simulink model "sixDOF6"  (R2024a)
settings: Solver=VariableStepAuto  StartTime=0.0  StopTime=30  MinStep=0.001  RelTol=1e-3
PreLoadFcn:
  | load("C:\Users\craig\OneDrive\Desktop\Matlab\TVC\Workspaces\rocketProps.mat");
undefined symbols (not defined in the file): magnitude, thrust, time
libraries: simulink x2, sharedtransform x2, aerolibanim x1, vrlib x1
settings Model: NumberOfSteps=100  Creator=craig  LastModifiedBy=craig
settings SolverCC: MaxConsecutiveMinStep=2
settings DebuggingCC: UnderSpecifiedDataTypeMsg=warning  UnderSpecifiedDimensionMsg=warning

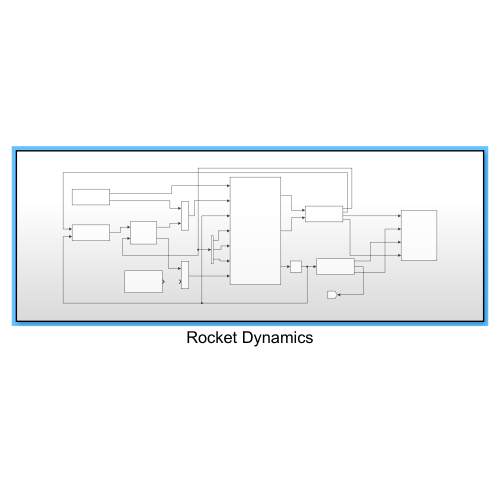
[thumbnail: Simulink's stored preview of the top-level diagram]
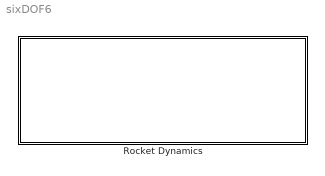
== system sixDOF6 ==
  Rocket Dynamics : Subsystem

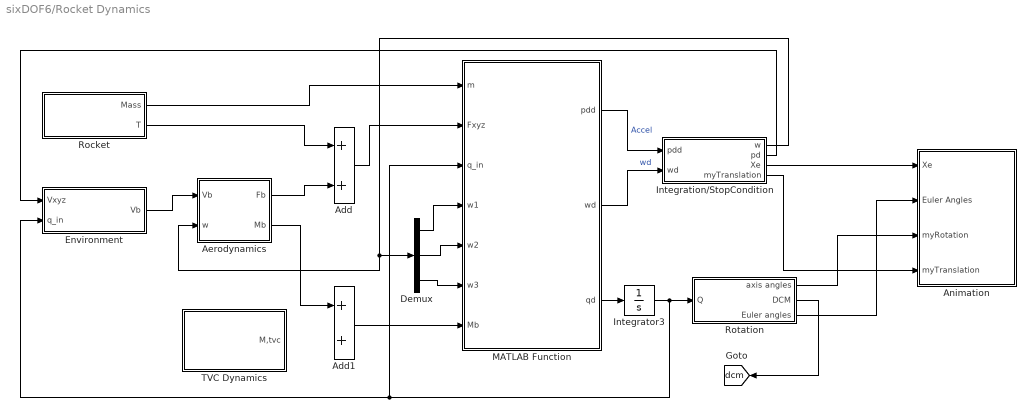
== system sixDOF6/Rocket Dynamics ==
  Add : Sum
  Add1 : Sum
  Aerodynamics : Subsystem
  Animation : Subsystem
  Demux : Demux  Outputs=3
  Environment : Subsystem
  Integration/StopCondition : Subsystem
  Integrator3 : Integrator  InitialCondition=[1; 0; 0; 0]
  MATLAB Function : MATLAB Function  TreatAsAtomicUnit=on
  Rocket : Subsystem
  Rotation : Subsystem
  TVC Dynamics : Subsystem
  tag scope: dcm=global
  wires:
  Integrator3/1 -> MATLAB Function/3(q_in), Environment/2(q_in), Rotation/1(Q)
  Add/1 -> MATLAB Function/2(Fxyz)
  Demux/1 -> MATLAB Function/4(w1)
  Environment/1("Vb ") -> Aerodynamics/1(Vb)
  Demux/3 -> MATLAB Function/6(w3)
  Aerodynamics/2(Mb) -> Add1/1
  Demux/2 -> MATLAB Function/5(w2)
  MATLAB Function/3(qd) -> Integrator3/1
  Rocket/2(T) -> Add/1
  Rocket/1(Mass) -> MATLAB Function/1(m)
  Aerodynamics/1(Fb) -> Add/2
  Rotation/2(DCM) -> [dcm]
  Add1/1 -> MATLAB Function/7(Mb)
  MATLAB Function/2(wd) -> Integration/StopCondition/2(wd)  "wd"
  Integration/StopCondition/1(w) -> Aerodynamics/2(w), Demux/1
  MATLAB Function/1(pdd) -> Integration/StopCondition/1(pdd)  "Accel"
  Integration/StopCondition/2(pd) -> Environment/1(Vxyz)
  Integration/StopCondition/3(Xe) -> Animation/1(Xe)
  Rotation/3(Euler angles) -> Animation/2(Euler Angles)
  Rotation/1(axis angles) -> Animation/3(myRotation)
  Integration/StopCondition/4(myTranslation) -> Animation/4(myTranslation)

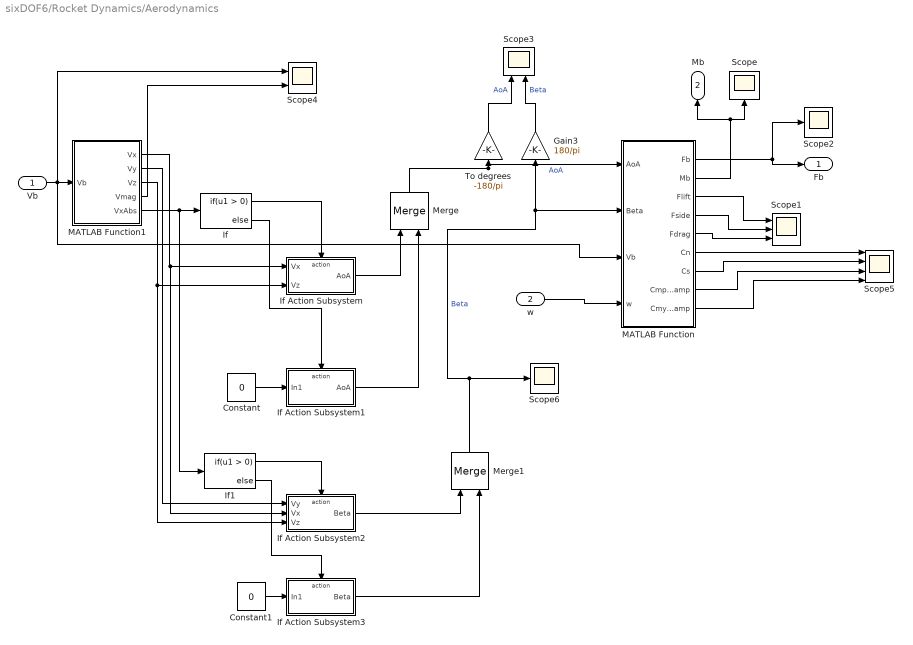
== system sixDOF6/Rocket Dynamics/Aerodynamics ==
  Vb : Inport
  w : Inport  Port=2
  Constant : Constant  Value=0
  Constant1 : Constant  Value=0
  Gain3 : Gain  Gain=180/pi
  If : If
  If Action Subsystem : Subsystem  TreatAsAtomicUnit=on
  If Action Subsystem1 : Subsystem  TreatAsAtomicUnit=on
  If Action Subsystem2 : Subsystem  TreatAsAtomicUnit=on
  If Action Subsystem3 : Subsystem  TreatAsAtomicUnit=on
  If1 : If
  MATLAB Function : MATLAB Function  TreatAsAtomicUnit=on
  MATLAB Function1 : MATLAB Function  TreatAsAtomicUnit=on
  Merge : Merge
  Merge1 : Merge
  Scope : Scope
  Scope1 : Scope  NumInputPorts=3
  Scope2 : Scope
  Scope3 : Scope  NumInputPorts=2
  Scope4 : Scope  NumInputPorts=2
  Scope5 : Scope  NumInputPorts=4
  Scope6 : Scope
  To degrees : Gain  Gain=-180/pi
  Fb : Outport
  Mb : Outport  Port=2
  wires:
  MATLAB Function/3(Flift) -> Scope1/1
  MATLAB Function/2(Mb) -> Scope/1, Mb/1
  MATLAB Function/1(Fb) -> Scope2/1, Fb/1
  MATLAB Function/5(Fdrag) -> Scope1/3
  Vb/1 -> Scope4/1, MATLAB Function/3(Vb), MATLAB Function1/1(Vb)
  If/2 -> If Action Subsystem1/Action
  Constant/1 -> If Action Subsystem1/1(In1)
  MATLAB Function1/1(Vx) -> If Action Subsystem2/2(Vx), If Action Subsystem/1(Vx)
  MATLAB Function1/3(Vz) -> If Action Subsystem2/3(Vz), If Action Subsystem/2(Vz)
  If/1 -> If Action Subsystem/Action
  If Action Subsystem/1(AoA) -> Merge/1
  If Action Subsystem1/1(AoA) -> Merge/2
  MATLAB Function1/2(Vy) -> If Action Subsystem2/1(Vy)
  Constant1/1 -> If Action Subsystem3/1(In1)
  If Action Subsystem2/1(Beta) -> Merge1/1
  If Action Subsystem3/1(Beta) -> Merge1/2
  If1/2 -> If Action Subsystem3/Action
  If1/1 -> If Action Subsystem2/Action
  MATLAB Function/4(Fside) -> Scope1/2
  Merge1/1 -> Scope6/1, Gain3/1, MATLAB Function/2(Beta)  "Beta"
  Merge/1 -> To degrees/1, MATLAB Function/1(AoA)  "AoA"
  MATLAB Function/6(Cn) -> Scope5/1
  MATLAB Function/7(Cs) -> Scope5/2
  Gain3/1 -> Scope3/2  "Beta"
  To degrees/1 -> Scope3/1  "AoA"
  MATLAB Function1/4(Vmag) -> Scope4/2
  MATLAB Function1/5(VxAbs) -> If1/1, If/1
  w/1 -> MATLAB Function/4(w)
  MATLAB Function/8(CmpDamp) -> Scope5/3
  MATLAB Function/9(CmyDamp) -> Scope5/4

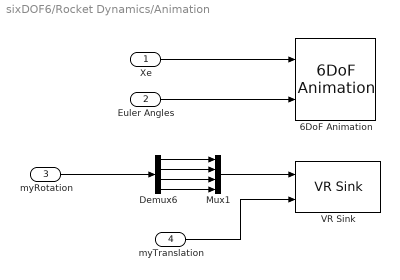
== system sixDOF6/Rocket Dynamics/Animation ==
  Xe : Inport
  Euler Angles : Inport  Port=2
  myRotation : Inport  Port=3
  myTranslation : Inport  Port=4
  6DoF Animation : aerolibanim/6DoF Animation  u1=[0 4000 -2000 2000 -5000 -3000]  u2=0.1  u3=100  u4=[4000 0 -5000]  u5=Fixed position  u6=[2000 500 -3150]  u7=10  u8=on
  Demux6 : Demux
  Mux1 : Mux
  VR Sink : vrlib/VR Sink  InstantiateOnLoad=on  SampleTime=0.1  ViewEnable=on  RemoteChange=off  RemoteView=off  FieldsWritten=MyTransform.rotation.4.1.1.double#MyTransform.translation.3.1.1.double  WorldFileName=C:\Users\craig\OneDrive\Desktop\Matlab\TVC\Animations\BestViewpoint.wrl  AutoView=off  VideoDimensions=[]  AllowVariableSize=off
  wires:
  Xe/1 -> 6DoF Animation/1
  Demux6/1 -> Mux1/1
  Demux6/3 -> Mux1/3
  myTranslation/1 -> VR Sink/2
  Demux6/2 -> Mux1/2
  Mux1/1 -> VR Sink/1
  myRotation/1 -> Demux6/1
  Demux6/4 -> Mux1/4
  Euler Angles/1 -> 6DoF Animation/2

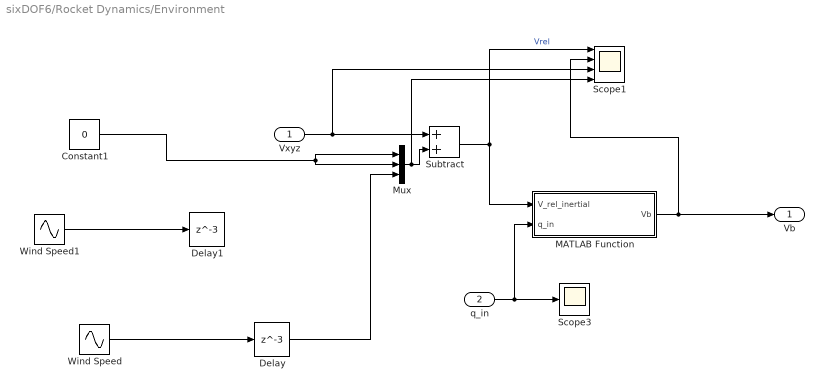
== system sixDOF6/Rocket Dynamics/Environment ==
  Vxyz : Inport
  q_in : Inport  Port=2
  Constant1 : Constant  Value=0
  Delay : Delay  DelayLength=3
  Delay1 : Delay  DelayLength=3
  MATLAB Function : MATLAB Function  TreatAsAtomicUnit=on
  Mux : Mux  Inputs=3
  Scope1 : Scope  NumInputPorts=4
  Scope3 : Scope
  Subtract : Sum
  Wind Speed : Sin  Amplitude=0.5  Bias=5  Frequency=2*pi*0.25  SampleTime=0
  Wind Speed1 : Sin  Amplitude=0.5  Bias=5  Frequency=2*pi*0.25  SampleTime=0
  "Vb " : Outport
  wires:
  Subtract/1 -> Scope1/1, MATLAB Function/1(V_rel_inertial)  "Vrel"
  Vxyz/1 -> Subtract/1, Scope1/3
  MATLAB Function/1(Vb) -> "Vb "/1, Scope1/2
  Constant1/1 -> Mux/1, Mux/2
  q_in/1 -> MATLAB Function/2(q_in), Scope3/1
  Mux/1 -> Scope1/4, Subtract/2
  Wind Speed1/1 -> Delay1/1
  Wind Speed/1 -> Delay/1
  Delay/1 -> Mux/3

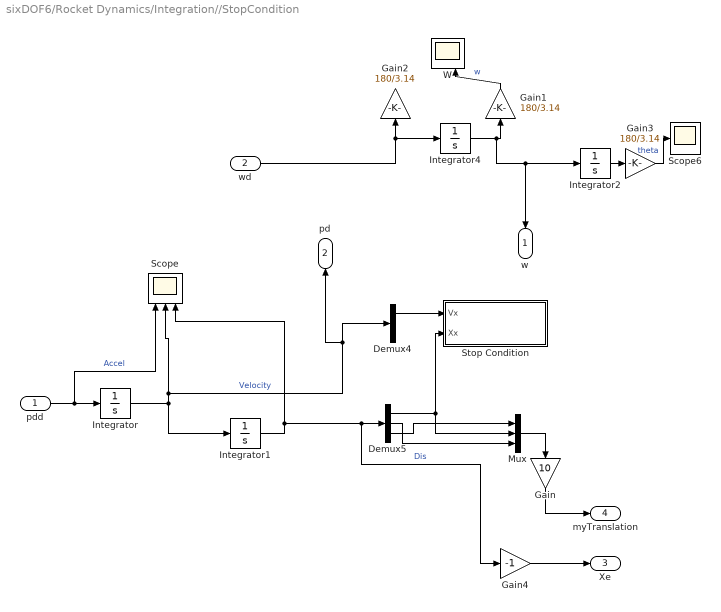
== system sixDOF6/Rocket Dynamics/Integration//StopCondition ==
  pdd : Inport
  wd : Inport  Port=2
  Demux4 : Demux  Outputs=3
  Demux5 : Demux  Outputs=3
  Gain : Gain  Gain=10
  Gain1 : Gain  Gain=180/3.14
  Gain2 : Gain  Gain=180/3.14
  Gain3 : Gain  Gain=180/3.14
  Gain4 : Gain  Gain=-1
  Integrator{,1..2,4} (4 alike) : Integrator  InitialCondition=[0; 0; 0]
  Mux : Mux  Inputs=3
  Scope : Scope  NumInputPorts=3
  Scope6 : Scope
  Stop Condition : Subsystem
  W : Scope  NumInputPorts=2
  w : Outport
  pd : Outport  Port=2
  Xe : Outport  Port=3
  myTranslation : Outport  Port=4
  wires:
  wd/1 -> Integrator4/1, Gain2/1
  Integrator2/1 -> Gain3/1
  Integrator4/1 -> w/1, Integrator2/1, Gain1/1
  Gain1/1 -> W/2  "w"
  Gain3/1 -> Scope6/1  "theta"
  Integrator/1 -> Integrator1/1, Demux4/1, pd/1, Scope/2  "Velocity"
  Demux5/3 -> Mux/1
  Demux5/2 -> Mux/3
  Demux4/1 -> Stop Condition/1(Vx)
  pdd/1 -> Scope/1, Integrator/1  "Accel"
  Gain4/1 -> Xe/1
  Integrator1/1 -> Scope/3, Gain4/1, Demux5/1  "Dis"
  Gain/1 -> myTranslation/1
  Mux/1 -> Gain/1
  Demux5/1 -> Stop Condition/2(Xx), Mux/2

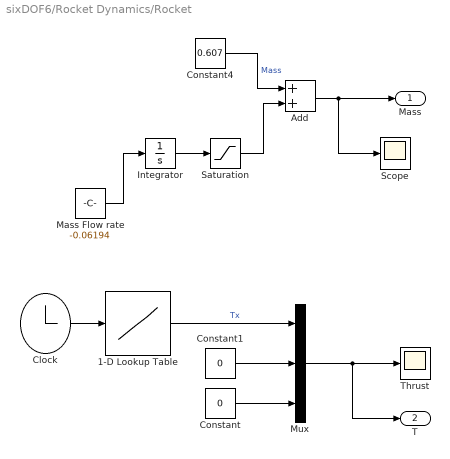
== system sixDOF6/Rocket Dynamics/Rocket ==
  1-D Lookup Table : Lookup_n-D  NumberOfTableDimensions=1  BreakpointsForDimension1=time  Table=thrust  TableMin=[0]  TableDataTypeStr=Inherit: Inherit from 'Table data'  ExtrapMethod=Clip  UseLastTableValue=on  InternalRulePriority=Speed  RndMeth=Simplest
  Add : Sum
  Clock : Clock
      settings: Decimation=100
  Constant : Constant  Value=0
  Constant1 : Constant  Value=0
  Constant4 : Constant  Value=0.607
  Integrator : Integrator  InitialCondition=0.188
  Mass Flow rate : Constant  Value=-0.06194
  Mux : Mux  Inputs=3
  Saturation : Saturate  LowerLimit=0.105
  Scope : Scope
  Thrust : Scope
  Mass : Outport
  T : Outport  Port=2
  wires:
  Clock/1 -> 1-D Lookup Table/1
  Constant1/1 -> Mux/2
  Mux/1 -> T/1, Thrust/1
  Constant4/1 -> Add/1  "Mass"
  Add/1 -> Scope/1, Mass/1
  1-D Lookup Table/1 -> Mux/1  "Tx"
  Constant/1 -> Mux/3
  Mass Flow rate/1 -> Integrator/1
  Integrator/1 -> Saturation/1
  Saturation/1 -> Add/2

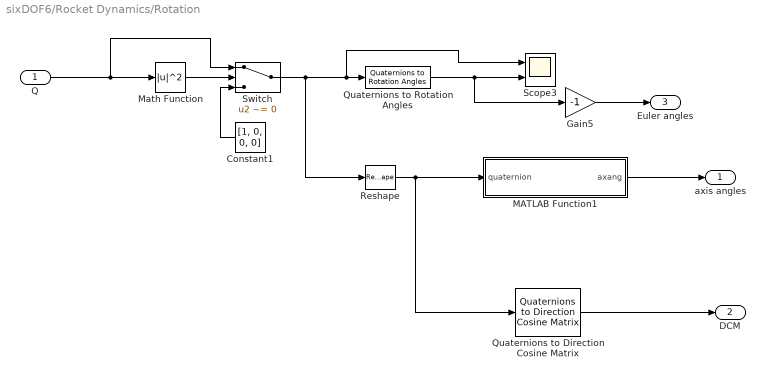
== system sixDOF6/Rocket Dynamics/Rotation ==
  Q : Inport
  Constant1 : Constant  Value=[1, 0, 0, 0]
  Gain5 : Gain  Gain=-1
  MATLAB Function1 : MATLAB Function  TreatAsAtomicUnit=on
  Math Function : Math  Operator=magnitude^2
  Quaternions to Direction Cosine Matrix : sharedtransform/Quaternions to  Direction Cosine Matrix  aMode=aMode
      settings: LibrarySourceBlock=|
      | aerolibtransform2/Quaternions to
      | Direction Cosine Matrix
  Quaternions to Rotation Angles : sharedtransform/Quaternions to Rotation Angles  rotationOrder=XYZ  aMode=aMode
  Reshape : Reshape  OutputDimensionality=Customize  OutputDimensions=[1,4]
  Scope3 : Scope  NumInputPorts=2
  Switch : Switch  Criteria=u2 ~= 0  SaturateOnIntegerOverflow=off  InputSameDT=off
  axis angles : Outport
  DCM : Outport  Port=2
  Euler angles : Outport  Port=3
  wires:
  Constant1/1 -> Switch/3
  Quaternions to Rotation Angles/1 -> Gain5/1, Scope3/2
  Switch/1 -> Reshape/1, Scope3/1, Quaternions to Rotation Angles/1
  Math Function/1 -> Switch/2
  Q/1 -> Switch/1, Math Function/1
  MATLAB Function1/1(axang) -> axis angles/1
  Reshape/1 -> Quaternions to Direction Cosine Matrix/1, MATLAB Function1/1(quaternion)
  Quaternions to Direction Cosine Matrix/1 -> DCM/1
  Gain5/1 -> Euler angles/1

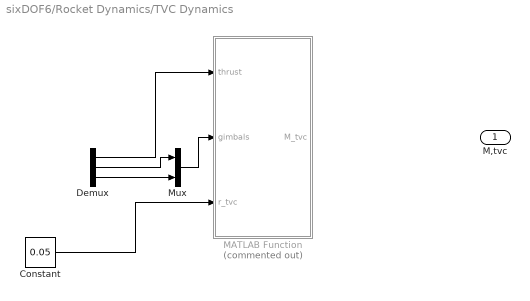
== system sixDOF6/Rocket Dynamics/TVC Dynamics ==
  Constant : Constant  Value=0.05
  Demux : Demux  Outputs=3
  MATLAB Function : MATLAB Function  Commented=on  TreatAsAtomicUnit=on
  Mux : Mux  Inputs=2
  M,tvc : Outport
  wires:
  Demux/1 -> MATLAB Function/1(thrust)
  Demux/2 -> Mux/1
  Demux/3 -> Mux/2
  Mux/1 -> MATLAB Function/2(gimbals)
  Constant/1 -> MATLAB Function/3(r_tvc)

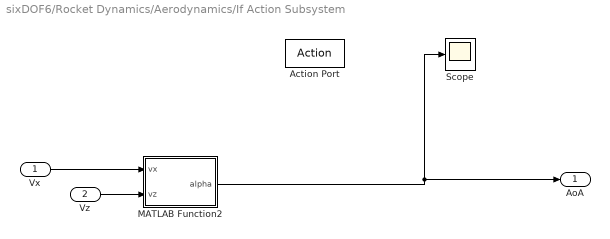
== system sixDOF6/Rocket Dynamics/Aerodynamics/If Action Subsystem ==
  Vx : Inport
  Vz : Inport  Port=2
  Action Port : ActionPort  ActionPortLabel=if(u1 > 0)
  MATLAB Function2 : MATLAB Function  TreatAsAtomicUnit=on
  Scope : Scope
  AoA : Outport
  wires:
  MATLAB Function2/1(alpha) -> Scope/1, AoA/1
  Vx/1 -> MATLAB Function2/1(vx)
  Vz/1 -> MATLAB Function2/2(vz)

== system sixDOF6/Rocket Dynamics/Aerodynamics/If Action Subsystem1 ==
  In1 : Inport
  Action Port : ActionPort  ActionPortLabel=else
  AoA : Outport
  wires:
  In1/1 -> AoA/1

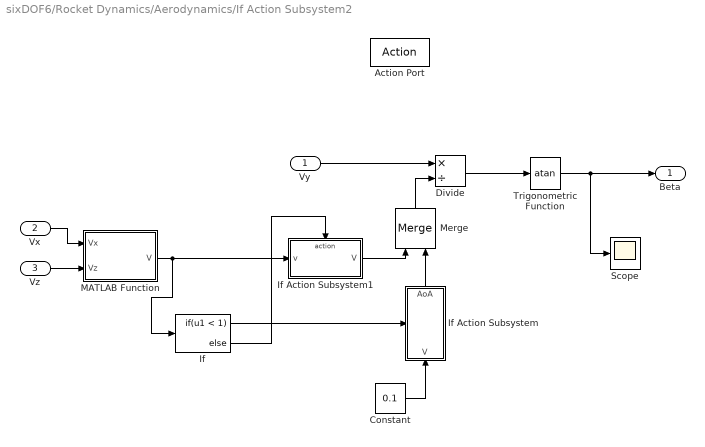
== system sixDOF6/Rocket Dynamics/Aerodynamics/If Action Subsystem2 ==
  Vy : Inport
  Vx : Inport  Port=2
  Vz : Inport  Port=3
  Action Port : ActionPort  ActionPortLabel=if(u1 > 0)
  Constant : Constant  Value=0.1
  Divide : Product  Inputs=*/
  If : If  IfExpression=u1 < 1
  If Action Subsystem : Subsystem  TreatAsAtomicUnit=on
  If Action Subsystem1 : Subsystem  TreatAsAtomicUnit=on
  MATLAB Function : MATLAB Function  TreatAsAtomicUnit=on
  Merge : Merge
  Scope : Scope
  Trigonometric Function : Trigonometry  Operator=atan
  Beta : Outport
  wires:
  Vx/1 -> MATLAB Function/1(Vx)
  Vz/1 -> MATLAB Function/2(Vz)
  Divide/1 -> Trigonometric Function/1
  Vy/1 -> Divide/1
  Constant/1 -> If Action Subsystem/1(V)
  Trigonometric Function/1 -> Scope/1, Beta/1
  If/1 -> If Action Subsystem/Action
  If Action Subsystem/1(AoA) -> Merge/2
  If/2 -> If Action Subsystem1/Action
  If Action Subsystem1/1(V) -> Merge/1
  Merge/1 -> Divide/2
  MATLAB Function/1(V) -> If/1, If Action Subsystem1/1(v)

== system sixDOF6/Rocket Dynamics/Aerodynamics/If Action Subsystem3 ==
  In1 : Inport
  Action Port : ActionPort  ActionPortLabel=else
  Beta : Outport
  wires:
  In1/1 -> Beta/1

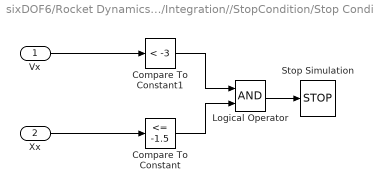
== system sixDOF6/Rocket Dynamics/Integration//StopCondition/Stop Condition ==
  Vx : Inport
  Xx : Inport  Port=2
  Compare To Constant : simulink/Logic and Bit Operations/Compare To Constant  relop=<=  const=-1.5  OutDataTypeStr=boolean
  Compare To Constant1 : simulink/Logic and Bit Operations/Compare To Constant  relop=<  const=-3  OutDataTypeStr=boolean
  Logical Operator : Logic  AllPortsSameDT=off  OutDataTypeStr=boolean
  Stop Simulation : Stop
  wires:
  Compare To Constant/1 -> Logical Operator/2
  Vx/1 -> Compare To Constant1/1
  Xx/1 -> Compare To Constant/1
  Compare To Constant1/1 -> Logical Operator/1
  Logical Operator/1 -> Stop Simulation/1

== system sixDOF6/Rocket Dynamics/Aerodynamics/If Action Subsystem2/If Action Subsystem ==
  V : Inport
  Action Port : ActionPort  ActionPortLabel=if(u1 < 1)
  AoA : Outport
  wires:
  V/1 -> AoA/1

== system sixDOF6/Rocket Dynamics/Aerodynamics/If Action Subsystem2/If Action Subsystem1 ==
  v : Inport
  Action Port : ActionPort  ActionPortLabel=else
  V : Outport
  wires:
  v/1 -> V/1

== matlab function sixDOF6/Rocket Dynamics/Aerodynamics/If Action Subsystem2/MATLAB Function ==
  data: Vx input; V output; Vz input
function V = fcn(Vx, Vz)

Vyz = [Vx; Vz];
V = norm(Vyz);

== matlab function sixDOF6/Rocket Dynamics/TVC Dynamics/MATLAB Function ==
  data: thrust input; M_tvc output; gimbals input; r_tvc input
function M_tvc = TVC_Controller(thrust, gimbals, r_tvc)


%TVC_Controller: Computes the thrust vector and the resulting moment

theta = gimbals(1);
psi = gimbals(2);

    % Define the thrust vector in the body frame
    TVC_body = thrust * [cos(theta) * cos(psi);  sin(psi); sin(theta)];
    
    % Calculate the moment arm (r_tvc cross T_body)
    M_tvc = cross(r_tvc, TVC_body);
    

end

== matlab function sixDOF6/Rocket Dynamics/Aerodynamics/If Action Subsystem/MATLAB Function2 ==
  data: vx input; alpha output; vz input
function alpha = fcn(vx, vz)

%if abs(vx) < 5
 %   alpha = 0;
%else
    alpha = atan2(vz, vx);
end

== matlab function sixDOF6/Rocket Dynamics/MATLAB Function ==
  data: m input; Fxyz input; q_in input size=4; w1 input; w2 input; w3 input; Mb input; pdd output size=[3,1]; wd output size=[3,1]; qd output
function [pdd, wd, qd] = EOM(m, Fxyz, q_in, w1, w2, w3, Mb)

q_in = q_in / norm(q_in); %normalise quaternion
Ix=0.00083;
Iy=0.00073;
Iz=0.00073;
g=9.81;
wx=w1;
wy=w2;
wz=w3;
w=[w1;w2;w3];

%Angular accelerations using newtons 2nd law for rotations in body frame
wxd = (1/Ix) * (Mb(1) + (Iy - Iz) * wy * wz);
wyd = (1/Iy) * (Mb(2) + (Iz - Ix) * wx * wz);
wzd = (1/Iz) * (Mb(3) + (Ix - Iy) * wx * wy);
wd =[wxd;wyd;wzd];


%update quaternion to reflect attitude change using formula for RoC of
%quaternion
qd=0.5*hamilton(q_in,[0;wx;wy;wz]);

% Net force from body to inertial frame
Fi_quat = hamilton(hamilton(q_in, [0; Fxyz]), conjugate(q_in));  % Reverse the order of quaternion transformation
Fi = Fi_quat(2:4); %remove scalar

% Translational accelerations
xdd = (Fi(1) / m) - g;
ydd = Fi(2) / m;      
zdd = (Fi(3) / m);    

pdd = [xdd; ydd; zdd];

function product = hamilton(q, r)
    product = [r(1)*q(1) - r(2)*q(2) - r(3)*q(3) - r(4)*q(4); 
               r(1)*q(2) + r(2)*q(1) + r(3)*q(4) - r(4)*q(3);
               r(1)*q(3) - r(2)*q(4) + r(3)*q(1) + r(4)*q(2);
               r(1)*q(4) + r(2)*q(3) - r(3)*q(2) + r(4)*q(1)];
end

%calculate conjugate of quaternion
    function q_star=conjugate(q)
        q_star=[q(1);-q(2);-q(3);-q(4)];
    end

end

== matlab function sixDOF6/Rocket Dynamics/Aerodynamics/MATLAB Function ==
  data: Fb output size=3; Mb output size=3; AoA input; Beta input; Flift output size=1; Fside output; Vb input size=3; Fdrag output size=3; Cn output; Cs output; w input; CmpDamp output; CmyDamp output
function [Fb, Mb, Flift, Fside, Fdrag, Cn, Cs, CmpDamp, CmyDamp] = Lift(AoA, Beta, Vb, w)
%define parameters
Ab = 0.003504635;
Afin = 0.00965;
Aplanform = 0.0835;
l = 0.202;
Mroll = 0;
rho = 1.225;
Cdx = 0.65;
d = 0.068;
Vbx = Vb(1);
Vby = Vb(2);
Vbz = Vb(3);
wy = w(2);
wz = w(3);
span = 0.1;
midchord = (90-85.134) * pi/180;
K = 1.1;

AoAThreshold = 5*pi/180;
Vmag = norm(Vb);
q = 0.5 * rho * norm(Vb)^2;
M = Vmag/340;
r = d/2;

%calculate Cn,Cs

if M > 1
    M = 0.99;%assuming Cn,Cs dont change with supersonic velocity
end

rho = span^2 * (1-M^2)^0.5 /Afin * cos(midchord); 

if abs(AoA) < AoAThreshold%account for nonlinear body lift aero affects over 5deg
    CnNose = 2 * sin(AoA)/Ab * pi * 0.229^2;
    Cnfins = 3 * (2*pi*span^2/Ab) / (1 + (1 + rho^2)^0.5);
    CnAoA = CnNose + Cnfins;
    Cn = CnAoA * -sin(AoA);
else
    CnNose = 2 * sin(AoA)/Ab * pi * 0.229^2;
    Cnfins = 3 * (2*pi*span^2/Ab)/ (1 + (1 + rho^2)^0.5);
    CnBodyLift = K * Aplanform/Ab * sin(AoA)^2;
    CnAoA = CnNose + Cnfins + CnBodyLift;
    Cn = CnAoA * -sin(AoA);%inversion to suit coord system
end
   
if abs(Beta) < AoAThreshold
    CsNose = 2 * sin(Beta)/Ab * pi * 0.229^2;
    Csfins = 3 * (2*pi*span^2/Ab)/ (1 + (1 + rho^2)^0.5);
    CsBeta = CsNose + Csfins;
    Cs = CsBeta * sin(Beta);
else
    CsNose = 2 * sin(Beta)/Ab * pi * 0.229^2;
    Csfins = 3 * (2*pi*span^2/Ab)/ (1 + (1 + rho^2)^0.5);
    CsBodyLift = K * Aplanform/Ab * sin(Beta)^2;
    CsBeta = CsNose + Csfins + CsBodyLift;
    Cs = CsBeta * sin(Beta);
end


%moment coefficients

Cmp = ((Cn * l)/d); %based of aoa 
Cmy = ((Cs * l)/d); %based of sideslip/beta

CmpDamp = -(1.25^4*r*-wy^2)/(Ab*d*Vmag^2);
CmyDamp = (1.25^4*r*-wz^2)/(Ab*d*Vmag^2);

Cmp = Cmp + CmpDamp;
Cmy = Cmy + CmyDamp;

% aero force vectors

if norm(Vb) > 1e-3
    Fdragmagx = q * Ab * Cdx; 
    Fdragx = Fdragmagx * (Vbx / norm(Vb) * sign(Vbx));
    Fdragyz = Fdragmagx * ([Vby*sign(Vby); Vbz*sign(Vbz)] / norm(Vb));
    Fdrag = [Fdragx; Fdragyz];
    Flift = q * Ab * Cn; %based off AoA
    Fside = q * Ab * Cs;  %based of sideslip/beta
    

    Mpitch = q * Ab * d * Cmp; %based of aoa 
    Myaw = q * Ab * d * Cmy; %based of sideslip/beta
   
else
   Fdrag = [0; 0; 0]; % No drag force when velocity is zero
   Flift = 0;  % No lift force when velocity is zero
   Fside = 0;  % No side force when velocity is zer0
  


   Mpitch = 0;
   Myaw = 0;
end


Fb =[0; -Fside; Flift] - Fdrag; %inversion for coord system ie y force induces z spin
Mb = [Mroll; -Mpitch; -Myaw];

end

== matlab function sixDOF6/Rocket Dynamics/Environment/MATLAB Function ==
  data: V_rel_inertial input; Vb output; q_in input size=4
function Vb = I_to_b(V_rel_inertial, q_in)

q_in = q_in / norm(q_in);

% Transform velocity to body frame quaternion using current orientation
Vb_quat = hamilton(hamilton(conjugate(q_in), [0; V_rel_inertial]), q_in);
Vb = Vb_quat(2:4);  % Remove scalar part



%calculate conjugate of quaternion
    function q_star=conjugate(q)
        q_star=[q(1);-q(2);-q(3);-q(4)];
    end

end

function product = hamilton(q, r)
    product = [r(1)*q(1) - r(2)*q(2) - r(3)*q(3) - r(4)*q(4);
               r(1)*q(2) + r(2)*q(1) + r(3)*q(4) - r(4)*q(3);
               r(1)*q(3) - r(2)*q(4) + r(3)*q(1) + r(4)*q(2);
               r(1)*q(4) + r(2)*q(3) - r(3)*q(2) + r(4)*q(1)];
end

== matlab function sixDOF6/Rocket Dynamics/Rotation/MATLAB Function1 ==
  data: quaternion input; axang output
function axang = fcn(quaternion)
    rotm = quat2rotm(quaternion);
   
    
%As rotm2axang outputs a 4 element vector including axis/angle together
    axang = -rotm2axang(rotm);
    
end

== matlab function sixDOF6/Rocket Dynamics/Aerodynamics/MATLAB Function1 ==
  data: Vx output; Vy output; Vz output; Vb input; Vmag output; VxAbs output
function [Vx, Vy, Vz, Vmag, VxAbs]= mag(Vb)

Vx = Vb(1);
Vy = Vb(2);
Vz = Vb(3);

VxAbs = abs(Vx);
Vmag = norm(Vb);

end
